simulink model "sgMdl_IO130_Loopback"  (R2024b)
settings: Solver=FixedStepAuto  StartTime=0.0  StopTime=inf  RelTol=1e-3  EnableMultiTasking=on
libraries: speedgoatlib_IO130 x3
Description:
  | IO130 - Analog Loopback
settings Model: sg_rtwmakecfg_data=_sglibc_  ModifiedByFormat=Speedgoat  Creator=Speedgoat  LastModifiedBy=Speedgoat
settings SolverCC: ConcurrentTasks=on  AlgebraicLoopSolver=TrustRegion  PositivePriorityOrder=on  AutoInsertRateTranBlk=on  InsertRTBMode=Never (minimum delay)
settings DataIOCC: SaveFormat=StructureWithTime  ReturnWorkspaceOutputs=off
settings OptimizationCC: BlockReduction=off  OptimizeBlockIOStorage=off  BufferReuse=off  GlobalBufferReuse=off  ExpressionFolding=off  LocalBlockOutputs=off
settings DebuggingCC: TasksWithSamePriorityMsg=none  UnconnectedInputMsg=warning  UnconnectedOutputMsg=warning  UnconnectedLineMsg=warning  SFExecutionAtInitializationDiag=none  ArithmeticOperatorsInVariantConditions=warning
settings HardwareCC: ProdBitPerLong=64  ProdLongLongMode=on  ProdHWDeviceType=Intel->x86-64 (Linux 64)
settings ModelReferenceCC: EnableRefExpFcnMdlSchedulingChecks=on
settings SFSimCC: SimUseLocalCustomCode=off  CustomCodeUndefinedFunction=UseInterfaceOnly
settings RTWCC: Description=Speedgoat Real-Time Target Machine  SystemTargetFile=speedgoat.tlc  TemplateMakefile=slrealtime_default_tmf  RTWUseLocalCustomCode=off  Toolchain=Simulink Real-Time Toolchain  BuildConfiguration=Faster Runs  TargetLang=C++  GPUComputeCapability=3.5  DLArmComputeVersion=19.05
settings CodeAppCC: StateflowObjectComments=on
settings SimulinkRealTimeTargetCC: SubcomponentCodeInterfacePackaging=Reusable function  InstructionSetFMA=off  LogToMDFFile=off  SLRTFileLogMaxRuns=10  UseGCCFastMath=on
settings ConfigComp: CovBoundaryAbsTol=1.0e-5

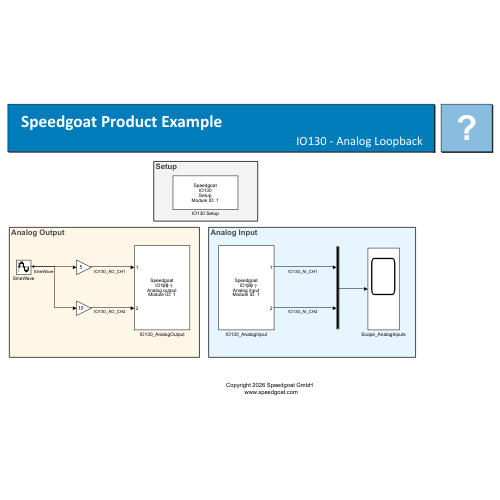
[thumbnail: Simulink's stored preview of the top-level diagram]
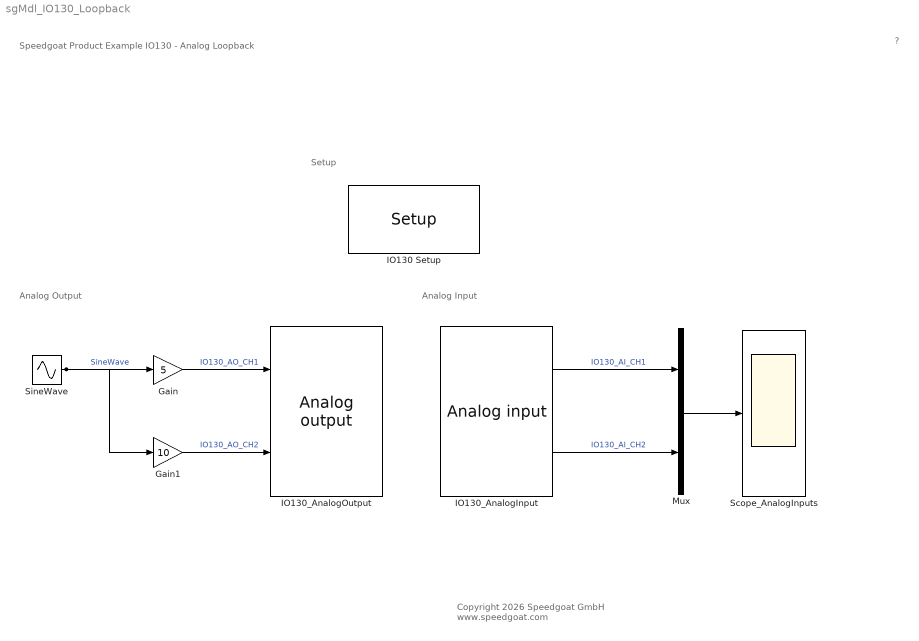
== system sgMdl_IO130_Loopback ==
  note: Setup
  note: Analog Output
  note: Analog Input
  note: Speedgoat Product Example
      | IO130 - Analog Loopback
  note: ?
  note: Copyright 2026 Speedgoat GmbH
      |  www.speedgoat.com
  Gain : Gain  Gain=5
  Gain1 : Gain  Gain=10
  IO130 Setup : speedgoatlib_IO130/Setup   parPciSlot=-1  parModuleId=1  parTriggerInitiator=Independent  parAdChannels=[1 2]  parAdRange=+-10V  parAdOversampling=None  parAdContinuousSampling=off  parAdDmaEn=off  parAdDisableCheck=off  parAdDmaChannels=All  parAdSampleClock=100e3  parAdDmaFrameSize=128  parAdSampleTime=-1  parDaChannels=[1 2]  parDaRange=+-10V  parDaInitValues=[0]  parDaResetValues=[1]  parDaDmaEn=off  parDaDisableCheck=off  parDaDmaChannels=All  parLatency=As small as possible  parDaSampleClock=100000  parClockLocked=on  parDaDmaFrameSize=128  parDaSampleTime=-1  parBoardType=130  parForceRefresh=11[]
      settings: SourceProductName=Simulink Real-Time: Speedgoat Library
  IO130_AnalogInput : speedgoatlib_IO130/Analog input   parModuleId=1  parSampleTime=0.001  parPciSlot=-1  parRange=+-10V  parOversampling=None  parChannels=[1 2]  parContinuousSampling=off  parDmaEn=off  parDmaChannels=All  parDmaConversionTime=1000  parDmaFrameSize=10  parBoardType=130  parIsInitialized=on
      settings: SourceProductName=Simulink Real-Time: Speedgoat Library
  IO130_AnalogOutput : speedgoatlib_IO130/Analog output   parModuleId=1  parSampleTime=0.001  parPciSlot=-1  parRange=+-10V  parChannels=[1 2]  parInitValues=[0 0]  parResetValues=[1 1]  parDmaChannels=All  parDmaEn=off  parDmaClkSrc=2  parDmaConversionTime=1000  parDmaFrameSize=10  parBoardType=130  parDoInterrupt=off  parLatency=As small as possible  parIsInitialized=on
      settings: SourceProductName=Simulink Real-Time: Speedgoat Library
  Mux : Mux  Inputs=2
  Scope_AnalogInputs : Scope
  SineWave : Sin  Frequency=2*pi  Samples=50  SampleTime=0.001
  wires:
  SineWave/1 -> Gain1/1, Gain/1  "SineWave"
  IO130_AnalogInput/1 -> Mux/1  "IO130_AI_CH1"
  IO130_AnalogInput/2 -> Mux/2  "IO130_AI_CH2"
  Mux/1 -> Scope_AnalogInputs/1
  Gain/1 -> IO130_AnalogOutput/1  "IO130_AO_CH1"
  Gain1/1 -> IO130_AnalogOutput/2  "IO130_AO_CH2"
